simulink model "state_fb_model_v3"  (R2019a)
settings: Solver=ode4  StartTime=0.0  StopTime=10  FixedStep=0.001  RelTol=1e-3
settings Model: Creator=chris  LastModifiedBy=chris

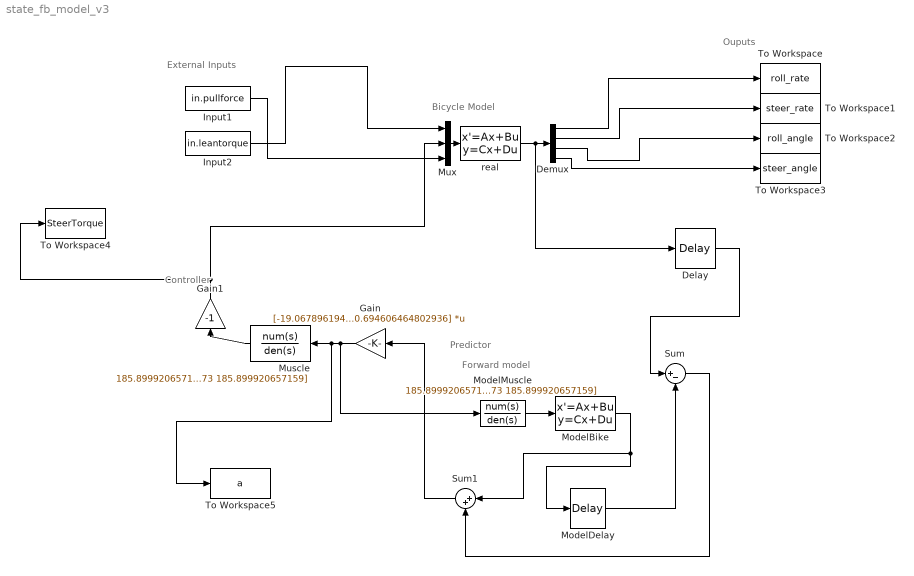
== system state_fb_model_v3 ==
  note: Bicycle Model
  note: External Inputs
  note: Controller
  note: Ouputs
  note: Predictor
  note: Forward model
  " ModelDelay " : TransportDelay  DelayTime=0.025
  Delay : TransportDelay  DelayTime=0.025
  Demux : Demux
  Gain : Gain  Gain=[-19.0678961940944 3.50720770775171 -3.42283102310238 0.694606464802936]  Multiplication=Matrix(K*u) (u vector)
  Gain1 : Gain  Gain=-1
  Input1 : FromWorkspace  VariableName=in.pullforce  SampleTime=0
  Input2 : FromWorkspace  VariableName=in.leantorque  SampleTime=0
  "ModelBike " : StateSpace  A=[-0.217084957502582 -0.732777146594285 7.84362144245841 -6.99366644658231;12.5140675589128 -10.9316923712887 18.9606745678989 17.2953442228593;1 0 0 0;0 1 0 0]  B=[-0.119659448859188;6.89788202882891;0;0]  C=[1 0 0 0;0 1 0 0;0 0 1 0;0 0 0 1]  D=[0;0;0;0]  InitialCondition=0
  ModelMuscle : TransferFcn  Numerator=185.899920657159  Denominator=[1 19.2821119516073 185.899920657159]
  Muscle : TransferFcn  Numerator=185.899920657159  Denominator=[1 19.2821119516073 185.899920657159]
  Mux : Mux  Inputs=3
  Sum : Sum  Inputs=|+-
  Sum1 : Sum  Inputs=|++
  To Workspace : ToWorkspace  VariableName=roll_rate  SampleTime=-1
  To Workspace1 : ToWorkspace  VariableName=steer_rate  SampleTime=-1
  To Workspace2 : ToWorkspace  VariableName=roll_angle  SampleTime=-1
  To Workspace3 : ToWorkspace  VariableName=steer_angle  SampleTime=-1
  To Workspace4 : ToWorkspace  VariableName=SteerTorque  SampleTime=-1
  To Workspace5 : ToWorkspace  VariableName=a  SampleTime=-1
  "real " : StateSpace  A=[-0.217084957502582 -0.732777146594285 7.84362144245841 -6.99366644658231;12.5140675589128 -10.9316923712887 18.9606745678989 17.2953442228593;1 0 0 0;0 1 0 0]  B=[0.00953456629028395 -0.119659448859188 0.00628498234467534;-0.119659448859188 6.89788202882891 -0.00112925277035058;0 0 0;0 0 0]  C=[1 0 0 0;0 1 0 0;0 0 1 0;0 0 0 1]  D=[0 0 0;0 0 0;0 0 0;0 0 0]  InitialCondition=0
  wires:
  Gain/1 -> ModelMuscle/1, To Workspace5/1, Muscle/1
  Gain1/1 -> Mux/2, To Workspace4/1
  Input1/1 -> Mux/3
  Mux/1 -> "real "/1
  Demux/1 -> To Workspace/1
  Demux/2 -> To Workspace1/1
  Demux/3 -> To Workspace2/1
  Demux/4 -> To Workspace3/1
  Input2/1 -> Mux/1
  Muscle/1 -> Gain1/1
  ModelMuscle/1 -> "ModelBike "/1
  Delay/1 -> Sum/1
  "ModelBike "/1 -> " ModelDelay "/1, Sum1/1
  " ModelDelay "/1 -> Sum/2
  Sum/1 -> Sum1/2
  Sum1/1 -> Gain/1
  "real "/1 -> Delay/1, Demux/1
